simulink model "PeakDetect_500"  (R2018b)
settings: Solver=FixedStepAuto  StartTime=0  StopTime=500*(15e-9)  FixedStep=15e-9  RelTol=1e-3
libraries: simulink x35, hdlsllib x34
(part 1 of 3)
settings Model: FPTRunName=FPA_Reference  Creator=jason  LastModifiedBy=jason
settings OptimizationCC: DefaultParameterBehavior=Inlined

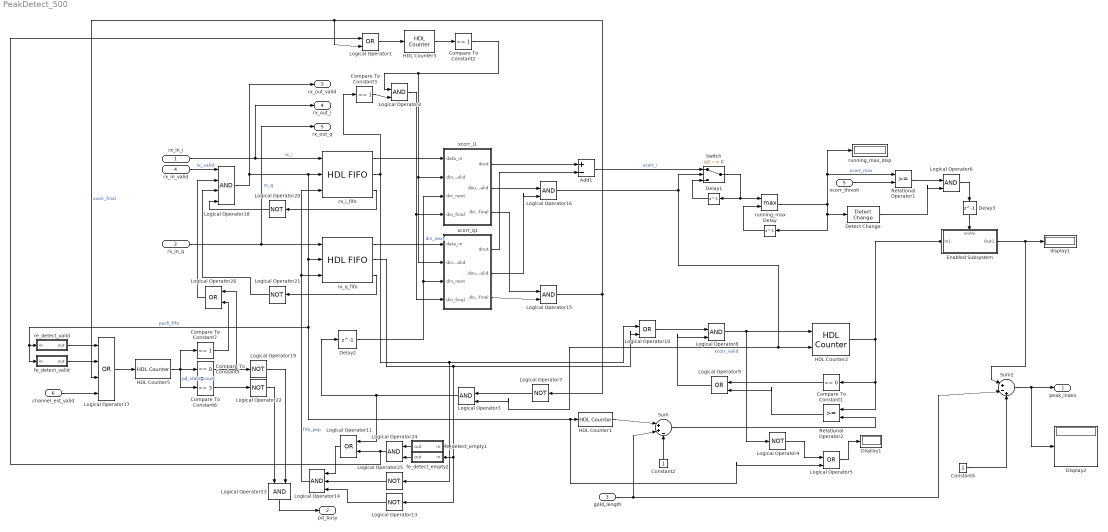
== system PeakDetect_500 ==
  rx_in_i : Inport  OutDataTypeStr=fixdt(1,16,15)  SampleTime=15e-9  Interpolate=off
  rx_in_q : Inport  Port=2  OutDataTypeStr=fixdt(1,16,15)  SampleTime=15e-9  Interpolate=off
  gold_length : Inport  Port=3  OutDataTypeStr=uint16  Interpolate=off
  rx_in_valid : Inport  Port=4  OutDataTypeStr=boolean  SampleTime=15e-9  Interpolate=off
  xcorr_thresh : Inport  Port=5  Interpolate=off
  channel_est_valid : Inport  Port=6  OutDataTypeStr=boolean  Interpolate=off
  Add1 : Sum  Inputs=+-
  Compare To Constant1 : simulink/Logic and Bit Operations/Compare To Constant  relop===  const=0  OutDataTypeStr=boolean
  Compare To Constant2 : simulink/Logic and Bit Operations/Compare To Constant  relop===  const=1  OutDataTypeStr=boolean
  Compare To Constant3 : simulink/Logic and Bit Operations/Compare To Constant  relop===  const=1  OutDataTypeStr=boolean
  Compare To Constant5 : simulink/Logic and Bit Operations/Compare To Constant  relop===  const=0  OutDataTypeStr=boolean
  Compare To Constant6 : simulink/Logic and Bit Operations/Compare To Constant  relop===  const=3  OutDataTypeStr=boolean
  Compare To Constant7 : simulink/Logic and Bit Operations/Compare To Constant  relop===  const=1  OutDataTypeStr=boolean
  Constant2 : Constant  OutDataTypeStr=uint8  SampleTime=-1
  Constant4 : Constant  OutDataTypeStr=uint16  SampleTime=-1
  Delay{,1..3} (4 alike) : Delay  DelayLength=1
  Detect Change : simulink/Logic and Bit Operations/Detect Change  vinit=0  OutDataTypeStr=boolean
  Display1 : Display
  Display2 : Display
  Enabled Subsystem : Subsystem  TreatAsAtomicUnit=on
  HDL Counter1 : hdlsllib/Sources/HDL Counter  CountType=Free running  CountInit=0  CountStep=1  CountMax=25  CountFromType=Initial value  CountFrom=0  CountResetPort=off  CountLoadPort=off  CountEnbPort=on  CountDirPort=off  CountDataType=Unsigned  CountWordLen=16  CountFracLen=0  CountSampTime=1
      settings: SourceProductBaseCode=HD
  HDL Counter2 : hdlsllib/Sources/HDL Counter  CountType=Free running  CountInit=0  CountStep=1  CountMax=25  CountFromType=Initial value  CountFrom=0  CountResetPort=on  CountLoadPort=off  CountEnbPort=on  CountDirPort=off  CountDataType=Unsigned  CountWordLen=16  CountFracLen=0  CountSampTime=1
      settings: SourceProductBaseCode=HD
  HDL Counter3 : hdlsllib/Sources/HDL Counter  CountType=Count limited  CountInit=0  CountStep=1  CountMax=1  CountFromType=Initial value  CountFrom=0  CountResetPort=off  CountLoadPort=off  CountEnbPort=on  CountDirPort=off  CountDataType=Unsigned  CountWordLen=4  CountFracLen=0  CountSampTime=1
      settings: SourceProductBaseCode=HD
  HDL Counter5 : hdlsllib/Sources/HDL Counter  CountType=Count limited  CountInit=0  CountStep=1  CountMax=3  CountFromType=Initial value  CountFrom=0  CountResetPort=off  CountLoadPort=off  CountEnbPort=on  CountDirPort=off  CountDataType=Unsigned  CountWordLen=4  CountFracLen=0  CountSampTime=1
      settings: SourceProductBaseCode=HD
  Logical Operator{1,5,9..11,26} (6 alike) : Logic  Operator=OR  IconShape=distinctive  AllPortsSameDT=off  OutDataTypeStr=boolean
  Logical Operator{4,7,13,19..22,25} (8 alike) : Logic  Operator=NOT  IconShape=distinctive  AllPortsSameDT=off  OutDataTypeStr=boolean
  Logical Operator14 : Logic  Inputs=3  IconShape=distinctive  AllPortsSameDT=off  OutDataTypeStr=boolean
  Logical Operator{2..3,6,8,15..16,23..24} (8 alike) : Logic  IconShape=distinctive  AllPortsSameDT=off  OutDataTypeStr=boolean
  Logical Operator17 : Logic  Operator=OR  Inputs=4  IconShape=distinctive  AllPortsSameDT=off  OutDataTypeStr=boolean
  Logical Operator18 : Logic  Inputs=4  IconShape=distinctive  AllPortsSameDT=off  OutDataTypeStr=boolean
  Relational Operator1 : RelationalOperator  OutDataTypeStr=boolean  RndMeth=Nearest
  Relational Operator2 : RelationalOperator  OutDataTypeStr=boolean  RndMeth=Nearest
  Sum : Sum  Inputs=|++-  AccumDataTypeStr=uint16
  Sum2 : Sum  Inputs=|+-+  AccumDataTypeStr=uint16
  Switch : Switch  Criteria=u2 ~= 0
  display1 : Display
  fe_detect_empty1 : Subsystem
  fe_detect_empty2 : Subsystem
  fe_detect_valid : Subsystem
  re_detect_valid : Subsystem
  running_max : MinMax  Function=max  Inputs=2
  running_max_disp : Display
  rx_i_fifo : hdlsllib/HDL RAMs/HDL FIFO  fifo_size=1024  ratio=1  push_msg=Warning  pop_msg=Warning  show_empty=on  show_full=on  show_num=off
      settings: SourceProductName=HDL Coder  SourceProductBaseCode=HD
  rx_q_fifo : hdlsllib/HDL RAMs/HDL FIFO  fifo_size=1024  ratio=1  push_msg=Warning  pop_msg=Warning  show_empty=on  show_full=on  show_num=off
      settings: SourceProductName=HDL Coder  SourceProductBaseCode=HD
  xcorr_i1 : Subsystem
  xcorr_q1 : Subsystem
  peak_index : Outport  OutDataTypeStr=uint16
  pd_busy : Outport  Port=2
  rx_out_valid : Outport  Port=3  SampleTime=15e-9
  rx_out_i : Outport  Port=4  SampleTime=15e-9
  rx_out_q : Outport  Port=5  SampleTime=15e-9
  wires:
  rx_in_i/1 -> rx_i_fifo/1, rx_out_i/1  "rx_i"
  Add1/1 -> Switch/1  "xcorr_i"
  Enabled Subsystem/1(Out1) -> display1/1, Sum2/1
  gold_length/1 -> Sum2/2, Sum/2
  Sum2/1 -> Display2/1, peak_index/1
  running_max/1 -> Relational Operator1/1, running_max_disp/1, Detect Change/1, Delay/1  "xcorr_max"
  Delay/1 -> running_max/2
  rx_in_q/1 -> rx_q_fifo/1, rx_out_q/1  "rx_q"
  rx_q_fifo/1 -> xcorr_q1/1(data_in)
  rx_i_fifo/2 -> Compare To Constant3/1, Logical Operator25/1, fe_detect_empty1/1(in), Logical Operator10/1
  rx_q_fifo/2 -> fe_detect_empty2/1(in), Logical Operator13/1, Logical Operator10/2
  Sum/1 -> Relational Operator2/2
  HDL Counter1/1 -> Sum/1
  Constant2/1 -> Sum/3
  Constant4/1 -> Sum2/3
  Logical Operator4/1 -> Logical Operator5/1
  Logical Operator5/1 -> Display1/1
  xcorr_thresh/1 -> Relational Operator1/2
  Relational Operator1/1 -> Logical Operator6/1
  Detect Change/1 -> Logical Operator6/2
  xcorr_i1/1(dout) -> Add1/1
  xcorr_q1/1(dout) -> Add1/2
  Logical Operator16/1 -> HDL Counter2/2, Logical Operator3/2, Switch/2  "xcorr_valid"
  HDL Counter2/1 -> Relational Operator2/1, Compare To Constant1/1, Enabled Subsystem/1(In1)
  Compare To Constant1/1 -> Logical Operator9/1
  Relational Operator2/1 -> Logical Operator9/2
  Logical Operator9/1 -> Logical Operator8/2
  Logical Operator8/1 -> Logical Operator4/1, HDL Counter2/1
  Logical Operator10/1 -> Logical Operator8/1
  Logical Operator3/1 -> Delay2/1, Logical Operator11/1
  Delay2/1 -> xcorr_i1/3(din_next), xcorr_q1/3(din_next)  "din_next"
  rx_i_fifo/1 -> xcorr_i1/1(data_in)
  Logical Operator6/1 -> Delay3/1
  Delay3/1 -> Enabled Subsystem/Enable
  HDL Counter3/1 -> Compare To Constant2/1
  Compare To Constant2/1 -> xcorr_i1/2(din_valid), xcorr_q1/2(din_valid), Logical Operator2/1
  Logical Operator24/1 -> Logical Operator1/1, Logical Operator11/2
  Logical Operator1/1 -> HDL Counter3/1
  Logical Operator15/1 -> Logical Operator7/1, Logical Operator17/3, Logical Operator1/2  "xcorr_final"
  Compare To Constant3/1 -> Logical Operator2/2
  Logical Operator2/1 -> xcorr_q1/4(din_final), xcorr_i1/4(din_final)
  Logical Operator7/1 -> Logical Operator3/1
  Logical Operator13/1 -> Logical Operator14/3
  Logical Operator11/1 -> Logical Operator14/1
  Logical Operator14/1 -> rx_i_fifo/3, rx_q_fifo/3  "fifo_pop"
  xcorr_i1/3(dout_final) -> Logical Operator15/1
  xcorr_q1/3(dout_final) -> Logical Operator15/2
  xcorr_q1/2(dout_valid) -> Logical Operator16/2
  xcorr_i1/2(dout_valid) -> Logical Operator16/1
  Logical Operator18/1 -> rx_out_valid/1, rx_q_fifo/2, Logical Operator5/2, HDL Counter1/1, fe_detect_valid/1(in), re_detect_valid/1(in), rx_i_fifo/2  "push_fifo"
  re_detect_valid/1(out) -> Logical Operator17/1
  fe_detect_valid/1(out) -> Logical Operator17/2
  Logical Operator17/1 -> HDL Counter5/1
  channel_est_valid/1 -> Logical Operator17/4
  HDL Counter5/1 -> Compare To Constant7/1, Compare To Constant6/1, Compare To Constant5/1  "pd_state_count"
  rx_in_valid/1 -> Logical Operator18/1  "rx_valid"
  rx_i_fifo/3 -> Logical Operator20/1
  rx_q_fifo/3 -> Logical Operator21/1
  Logical Operator21/1 -> Logical Operator18/3
  Logical Operator20/1 -> Logical Operator18/4
  Compare To Constant5/1 -> Logical Operator26/1, Logical Operator19/1
  Compare To Constant6/1 -> Logical Operator22/1
  Logical Operator22/1 -> Logical Operator23/1
  Logical Operator19/1 -> Logical Operator23/2
  Logical Operator23/1 -> pd_busy/1
  fe_detect_empty1/1(out) -> Logical Operator24/1
  fe_detect_empty2/1(out) -> Logical Operator24/2
  Logical Operator25/1 -> Logical Operator14/2
  Logical Operator26/1 -> Logical Operator18/2
  Compare To Constant7/1 -> Logical Operator26/2
  Switch/1 -> Delay1/1, running_max/1
  Delay1/1 -> Switch/3

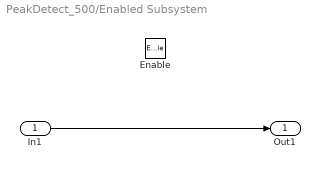
== system PeakDetect_500/Enabled Subsystem ==
  In1 : Inport
  Enable : EnablePort
  Out1 : Outport  InitialOutput=0
  wires:
  In1/1 -> Out1/1

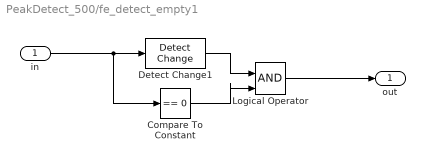
== system PeakDetect_500/fe_detect_empty1 ==
  in : Inport  OutDataTypeStr=boolean
  Compare To Constant : simulink/Logic and Bit Operations/Compare To Constant  relop===  const=0  OutDataTypeStr=boolean
  Detect Change1 : simulink/Logic and Bit Operations/Detect Change  vinit=0  OutDataTypeStr=boolean
  Logical Operator : Logic  IconShape=distinctive  AllPortsSameDT=off  OutDataTypeStr=boolean
  out : Outport  OutDataTypeStr=boolean
  wires:
  Logical Operator/1 -> out/1
  Detect Change1/1 -> Logical Operator/1
  Compare To Constant/1 -> Logical Operator/2
  in/1 -> Compare To Constant/1, Detect Change1/1

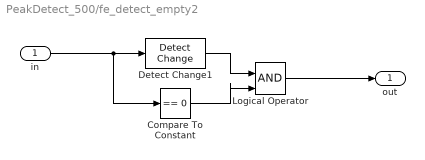
== system PeakDetect_500/fe_detect_empty2 ==
  in : Inport  OutDataTypeStr=boolean
  Compare To Constant : simulink/Logic and Bit Operations/Compare To Constant  relop===  const=0  OutDataTypeStr=boolean
  Detect Change1 : simulink/Logic and Bit Operations/Detect Change  vinit=0  OutDataTypeStr=boolean
  Logical Operator : Logic  IconShape=distinctive  AllPortsSameDT=off  OutDataTypeStr=boolean
  out : Outport  OutDataTypeStr=boolean
  wires:
  Logical Operator/1 -> out/1
  Detect Change1/1 -> Logical Operator/1
  Compare To Constant/1 -> Logical Operator/2
  in/1 -> Compare To Constant/1, Detect Change1/1

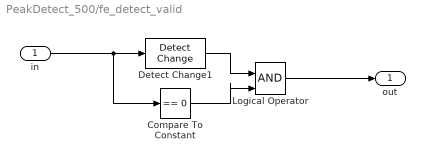
== system PeakDetect_500/fe_detect_valid ==
  in : Inport  OutDataTypeStr=boolean
  Compare To Constant : simulink/Logic and Bit Operations/Compare To Constant  relop===  const=0  OutDataTypeStr=boolean
  Detect Change1 : simulink/Logic and Bit Operations/Detect Change  vinit=0  OutDataTypeStr=boolean
  Logical Operator : Logic  IconShape=distinctive  AllPortsSameDT=off  OutDataTypeStr=boolean
  out : Outport  OutDataTypeStr=boolean
  wires:
  Logical Operator/1 -> out/1
  Detect Change1/1 -> Logical Operator/1
  Compare To Constant/1 -> Logical Operator/2
  in/1 -> Compare To Constant/1, Detect Change1/1

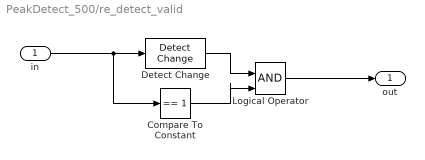
== system PeakDetect_500/re_detect_valid ==
  in : Inport  OutDataTypeStr=boolean
  Compare To Constant : simulink/Logic and Bit Operations/Compare To Constant  relop===  const=1  OutDataTypeStr=boolean
  Detect Change : simulink/Logic and Bit Operations/Detect Change  vinit=0  OutDataTypeStr=boolean
  Logical Operator : Logic  IconShape=distinctive  AllPortsSameDT=off  OutDataTypeStr=boolean
  out : Outport  OutDataTypeStr=boolean
  wires:
  Logical Operator/1 -> out/1
  Compare To Constant/1 -> Logical Operator/2
  Detect Change/1 -> Logical Operator/1
  in/1 -> Compare To Constant/1, Detect Change/1

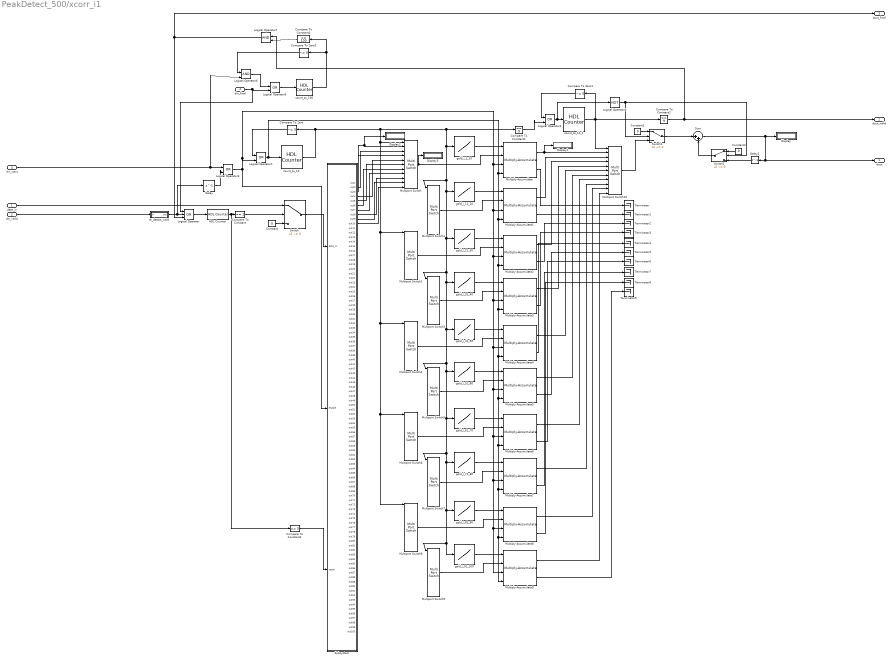
== system PeakDetect_500/xcorr_i1 ==
  data_in : Inport  OutDataTypeStr=fixdt(1,16,15)
  din_valid : Inport  Port=2
  din_next : Inport  Port=3
  din_final : Inport  Port=4
  Compare To Constant : simulink/Logic and Bit Operations/Compare To Constant  relop===  const=1  OutDataTypeStr=boolean
  Compare To Constant1 : simulink/Logic and Bit Operations/Compare To Constant  relop===  const=9  OutDataTypeStr=boolean
  Compare To Constant2 : simulink/Logic and Bit Operations/Compare To Constant  relop===  const=9  OutDataTypeStr=boolean
  Compare To Constant3 : simulink/Logic and Bit Operations/Compare To Constant  relop===  const=100  OutDataTypeStr=boolean
  Compare To Constant4 : simulink/Logic and Bit Operations/Compare To Constant  relop===  const=0  OutDataTypeStr=boolean
  Compare To Zero : simulink/Logic and Bit Operations/Compare To Zero  relop=~=  OutDataTypeStr=boolean
  Compare To Zero1 : simulink/Logic and Bit Operations/Compare To Zero  relop=~=  OutDataTypeStr=boolean
  Compare To Zero2 : simulink/Logic and Bit Operations/Compare To Zero  relop=~=  OutDataTypeStr=boolean
  Constant : Constant  Value=0  OutDataTypeStr=fixdt(1,16,15)  SampleTime=-1
  Constant1 : Constant  Value=0  OutDataTypeStr=Inherit: Inherit via back propagation  SampleTime=-1
  Constant2 : Constant  Value=0  OutDataTypeStr=Inherit: Inherit via back propagation  SampleTime=-1
  Delay : Delay  DelayLength=1
  Delay2 : Delay  DelayLength=1
  Display{,1..3} (4 alike) : Display
  HDL Counter : hdlsllib/Sources/HDL Counter  CountType=Count limited  CountInit=0  CountStep=1  CountMax=2  CountFromType=Initial value  CountFrom=0  CountResetPort=off  CountLoadPort=off  CountEnbPort=on  CountDirPort=off  CountDataType=Unsigned  CountWordLen=8  CountFracLen=0  CountSampTime=1
      settings: SourceProductBaseCode=HD
  Logical Operator : Logic  Operator=OR  Inputs=3  IconShape=distinctive  AllPortsSameDT=off  OutDataTypeStr=boolean
  Logical Operator{1..3,5} (4 alike) : Logic  Operator=OR  IconShape=distinctive  AllPortsSameDT=off  OutDataTypeStr=boolean
  Logical Operator4 : Logic  Operator=NOT  IconShape=distinctive  AllPortsSameDT=off  OutDataTypeStr=boolean
  Logical Operator6 : Logic  IconShape=distinctive  AllPortsSameDT=off  OutDataTypeStr=boolean
  Logical Operator7 : Logic  IconShape=distinctive  AllPortsSameDT=off  OutDataTypeStr=boolean
  Multiply-Accumulate{,1..9} (10 alike) : hdlsllib/HDL Operations/Multiply-Accumulate  opMode=Streaming - using Start and End ports  initValueSetting=Dialog  initValue=0  initValueSetting2=Dialog  initValue2=0  initValueSetting3=Dialog  initValue3=0  num_samples=2  RndMeth2=Floor  RndMeth3=Floor  datatype2=fixdt(1,32,16)  datatype3=Inherit: Inherit via back propagation  validOut=on  endInandOut=off  startOut=off  countOut=on  dim=-1  DoSatur=off  parallel=off
      settings: SourceProductName=HDL Coder  SourceProductBaseCode=HD
  Multiport Switch{,1..9} (10 alike) : MultiPortSwitch  DataPortOrder=Zero-based contiguous  Inputs=10  zeroidx=on  OutDataTypeStr=fixdt(1,16,15)
  Multiport Switch10 : MultiPortSwitch  DataPortOrder=Zero-based contiguous  Inputs=10  zeroidx=on  OutDataTypeStr=fixdt(1,32,16)
  Subsystem : Subsystem
  Sum : Sum  Inputs=|++  OutDataTypeStr=Inherit: Inherit via back propagation
  Switch : Switch  Criteria=u2 ~= 0  OutDataTypeStr=Inherit: Inherit via back propagation
  Switch1 : Switch  Criteria=u2 ~= 0  OutDataTypeStr=Inherit: Inherit via back propagation
  Switch2 : Switch  Criteria=u2 ~= 0  OutDataTypeStr=Inherit: Inherit via back propagation
  Terminator{,1..9} (10 alike) : Terminator
  count_to_10 : hdlsllib/Sources/HDL Counter  CountType=Count limited  CountInit=0  CountStep=1  CountMax=9  CountFromType=Initial value  CountFrom=0  CountResetPort=off  CountLoadPort=off  CountEnbPort=on  CountDirPort=off  CountDataType=Unsigned  CountWordLen=4  CountFracLen=0  CountSampTime=1
      settings: SourceProductBaseCode=HD
  count_to_100 : hdlsllib/Sources/HDL Counter  CountType=Count limited  CountInit=0  CountStep=1  CountMax=100  CountFromType=Initial value  CountFrom=0  CountResetPort=off  CountLoadPort=off  CountEnbPort=on  CountDirPort=off  CountDataType=Unsigned  CountWordLen=8  CountFracLen=0  CountSampTime=1
      settings: SourceProductBaseCode=HD
  count_to_10_2 : hdlsllib/Sources/HDL Counter  CountType=Count limited  CountInit=0  CountStep=1  CountMax=9  CountFromType=Initial value  CountFrom=0  CountResetPort=off  CountLoadPort=off  CountEnbPort=on  CountDirPort=off  CountDataType=Unsigned  CountWordLen=4  CountFracLen=0  CountSampTime=1
      settings: SourceProductBaseCode=HD
  gold_i_11_20 : Lookup_n-D  NumberOfTableDimensions=1  LookupTableObject=''  BreakpointsForDimension1=uint8([0,1,2,3,4,5,6,7,8,9])  BreakpointsForDimension1FirstPoint=10  BreakpointsForDimension2FirstPoint=10  BreakpointsForDimension1Spacing=12  BreakpointsForDimension2Spacing=12  IndexSearchMethod=Evenly spaced points  Table=|  TableDataTypeStr=fixdt(1,16,15)  InterpMethod=Flat  DiagnosticForOutOfRangeInput=Error  InternalRulePriority=Speed  OutDataTypeStr=fixdt(1,16,15)  RndMeth=Simplest  InputSameDT=on
      | [0.236906374990369
      | 0.265062589296935
      | 0.290853922757752
      | 0.306866645010829
      | 0.306877356493505
      | 0.282583044796408
      | 0.237895318583737
      | 0.179451570247324
      | 0.106711739895776
      | 0.0250742736874029]
  gold_i_1_10 : Lookup_n-D  NumberOfTableDimensions=1  LookupTableObject=''  BreakpointsForDimension1=uint8([0,1,2,3,4,5,6,7,8,9])  BreakpointsForDimension1FirstPoint=10  BreakpointsForDimension2FirstPoint=10  BreakpointsForDimension1Spacing=12  BreakpointsForDimension2Spacing=12  IndexSearchMethod=Evenly spaced points  Table=|  TableDataTypeStr=fixdt(1,16,15)  InterpMethod=Flat  DiagnosticForOutOfRangeInput=Error  InternalRulePriority=Speed  OutDataTypeStr=fixdt(1,16,15)  RndMeth=Simplest  InputSameDT=on
      | [0.357169275362262
      | 0.373691122276015
      | 0.363136475782144
      | 0.332586509539436
      | 0.291374087870011
      | 0.249422279627694
      | 0.215579045674242
      | 0.200455944131648
      | 0.201796906991478
      | 0.213779029408702]
  gold_i_21_30 : Lookup_n-D  NumberOfTableDimensions=1  LookupTableObject=''  BreakpointsForDimension1=uint8([0,1,2,3,4,5,6,7,8,9])  BreakpointsForDimension1FirstPoint=10  BreakpointsForDimension2FirstPoint=10  BreakpointsForDimension1Spacing=12  BreakpointsForDimension2Spacing=12  IndexSearchMethod=Evenly spaced points  Table=|  TableDataTypeStr=fixdt(1,16,15)  InterpMethod=Flat  DiagnosticForOutOfRangeInput=Error  InternalRulePriority=Speed  OutDataTypeStr=fixdt(1,16,15)  RndMeth=Simplest  InputSameDT=on
      | [-0.0591515848508664
      | -0.139598314313151
      | -0.210629837752387
      | -0.263713716480122
      | -0.301489962058033
      | -0.328238114626508
      | -0.340130412877520
      | -0.338689881672749
      | -0.326243180584237
      | -0.305614110780615]
  gold_i_31_40 : Lookup_n-D  NumberOfTableDimensions=1  LookupTableObject=''  BreakpointsForDimension1=uint8([0,1,2,3,4,5,6,7,8,9])  BreakpointsForDimension1FirstPoint=10  BreakpointsForDimension2FirstPoint=10  BreakpointsForDimension1Spacing=12  BreakpointsForDimension2Spacing=12  IndexSearchMethod=Evenly spaced points  Table=|  TableDataTypeStr=fixdt(1,16,15)  InterpMethod=Flat  DiagnosticForOutOfRangeInput=Error  InternalRulePriority=Speed  OutDataTypeStr=fixdt(1,16,15)  RndMeth=Simplest  InputSameDT=on
      | [-0.279858098355888
      | -0.247814863771713
      | -0.225446174923891
      | -0.202743193363060
      | -0.186527042991191
      | -0.178781266249413
      | -0.180711431323688
      | -0.192575241083779
      | -0.213551675353352
      | -0.245925394077466]
  gold_i_41_50 : Lookup_n-D  NumberOfTableDimensions=1  LookupTableObject=''  BreakpointsForDimension1=uint8([0,1,2,3,4,5,6,7,8,9])  BreakpointsForDimension1FirstPoint=10  BreakpointsForDimension2FirstPoint=10  BreakpointsForDimension1Spacing=12  BreakpointsForDimension2Spacing=12  IndexSearchMethod=Evenly spaced points  Table=|  TableDataTypeStr=fixdt(1,16,15)  InterpMethod=Flat  DiagnosticForOutOfRangeInput=Error  InternalRulePriority=Speed  OutDataTypeStr=fixdt(1,16,15)  RndMeth=Simplest  InputSameDT=on
      | [-0.273649789754997
      | -0.305507933389466
      | -0.332526349511340
      | -0.349961882407133
      | -0.353614169955030
      | -0.340366684130075
      | -0.308641627170326
      | -0.254460428744123
      | -0.185247665828561
      | -0.110080691949015]
  gold_i_51_60 : Lookup_n-D  NumberOfTableDimensions=1  LookupTableObject=''  BreakpointsForDimension1=uint8([0,1,2,3,4,5,6,7,8,9])  BreakpointsForDimension1FirstPoint=10  BreakpointsForDimension2FirstPoint=10  BreakpointsForDimension1Spacing=12  BreakpointsForDimension2Spacing=12  IndexSearchMethod=Evenly spaced points  Table=|  TableDataTypeStr=fixdt(1,16,15)  InterpMethod=Flat  DiagnosticForOutOfRangeInput=Error  InternalRulePriority=Speed  OutDataTypeStr=fixdt(1,16,15)  RndMeth=Simplest  InputSameDT=on
      | [-0.0297558495000080
      | 0.0499350486257353
      | 0.122950591883728
      | 0.183532283875116
      | 0.226715241693549
      | 0.244522518247979
      | 0.247772413924009
      | 0.223279362418140
      | 0.176793915855740
      | 0.111355596734925]
  gold_i_61_70 : Lookup_n-D  NumberOfTableDimensions=1  LookupTableObject=''  BreakpointsForDimension1=uint8([0,1,2,3,4,5,6,7,8,9])  BreakpointsForDimension1FirstPoint=10  BreakpointsForDimension2FirstPoint=10  BreakpointsForDimension1Spacing=12  BreakpointsForDimension2Spacing=12  IndexSearchMethod=Evenly spaced points  Table=|  TableDataTypeStr=fixdt(1,16,15)  InterpMethod=Flat  DiagnosticForOutOfRangeInput=Error  InternalRulePriority=Speed  OutDataTypeStr=fixdt(1,16,15)  RndMeth=Simplest  InputSameDT=on
      | [0.0312880626224120
      | -0.0580988665112754
      | -0.150830519884918
      | -0.236354458852815
      | -0.321361371110983
      | -0.387151947785857
      | -0.432910784333285
      | -0.454553321854592
      | -0.449340647995132
      | -0.416266380216616]
  gold_i_71_80 : Lookup_n-D  NumberOfTableDimensions=1  LookupTableObject=''  BreakpointsForDimension1=uint8([0,1,2,3,4,5,6,7,8,9])  BreakpointsForDimension1FirstPoint=10  BreakpointsForDimension2FirstPoint=10  BreakpointsForDimension1Spacing=12  BreakpointsForDimension2Spacing=12  IndexSearchMethod=Evenly spaced points  Table=|  TableDataTypeStr=fixdt(1,16,15)  InterpMethod=Flat  DiagnosticForOutOfRangeInput=Error  InternalRulePriority=Speed  OutDataTypeStr=fixdt(1,16,15)  RndMeth=Simplest  InputSameDT=on
      | [-0.356405677154333
      | -0.268905527196357
      | -0.172503144328213
      | -0.0623088722264564
      | 0.0478292512438747
      | 0.147701871156711
      | 0.227579808283800
      | 0.279365016179912
      | 0.297653875710057
      | 0.276310228166542]
  gold_i_81_90 : Lookup_n-D  NumberOfTableDimensions=1  LookupTableObject=''  BreakpointsForDimension1=uint8([0,1,2,3,4,5,6,7,8,9])  BreakpointsForDimension1FirstPoint=10  BreakpointsForDimension2FirstPoint=10  BreakpointsForDimension1Spacing=12  BreakpointsForDimension2Spacing=12  IndexSearchMethod=Evenly spaced points  Table=|  TableDataTypeStr=fixdt(1,16,15)  InterpMethod=Flat  DiagnosticForOutOfRangeInput=Error  InternalRulePriority=Speed  OutDataTypeStr=fixdt(1,16,15)  RndMeth=Simplest  InputSameDT=on
      | [0.222595237130309
      | 0.147485843722747
      | 0.0555170073150737
      | -0.0424496465550990
      | -0.134707118174198
      | -0.210100315272752
      | -0.259403813850479
      | -0.272248751146779
      | -0.259403813850479
      | -0.210100315272752]
  gold_i_91_100 : Lookup_n-D  NumberOfTableDimensions=1  LookupTableObject=''  BreakpointsForDimension1=uint8([0,1,2,3,4,5,6,7,8,9])  BreakpointsForDimension1FirstPoint=10  BreakpointsForDimension2FirstPoint=10  BreakpointsForDimension1Spacing=12  BreakpointsForDimension2Spacing=12  IndexSearchMethod=Evenly spaced points  Table=|  TableDataTypeStr=fixdt(1,16,15)  InterpMethod=Flat  DiagnosticForOutOfRangeInput=Error  InternalRulePriority=Speed  OutDataTypeStr=fixdt(1,16,15)  RndMeth=Simplest  InputSameDT=on
      | [-0.134707118174198
      | -0.0424496465550990
      | 0.0555170073150737
      | 0.147485843722747
      | 0.222595237130309
      | 0.267820298855522
      | 0.290378842162360
      | 0.275261187855880
      | 0.228204197191429
      | 0.153805243290024]
  re_detect_valid : Subsystem
  dout : Outport  OutDataTypeStr=fixdt(1,32,16)
  dout_valid : Outport  Port=2
  dout_final : Outport  Port=3
  wires:
  ? -> Multiport Switch3/4
  Compare To Constant2/1 -> dout_valid/1, Logical Operator7/1
  ? -> Multiport Switch4/6
  ? -> Multiport Switch1/8
  Logical Operator1/1 -> count_to_10/1, Multiply-Accumulate2/4, Multiply-Accumulate9/4, Multiply-Accumulate8/4, Multiply-Accumulate7/4, Multiply-Accumulate6/4, Multiply-Accumulate5/4, Multiply-Accumulate4/4, Multiply-Accumulate3/4, Multiply-Accumulate1/4, Multiply-Accumulate/4
  gold_i_21_30/1 -> Multiply-Accumulate2/1
  HDL Counter/1 -> Compare To Constant4/1, Compare To Constant/1
  count_to_100/1 -> Compare To Constant3/1, Compare To Zero2/1
  Subsystem/5(out5) -> Multiport Switch/6
  Logical Operator3/1 -> Subsystem/2(enable), Multiply-Accumulate9/3, Multiply-Accumulate8/3, Multiply-Accumulate7/3, Multiply-Accumulate6/3, Multiply-Accumulate5/3, Multiply-Accumulate4/3, Multiply-Accumulate3/3, Multiply-Accumulate2/3, Multiply-Accumulate1/3, Multiply-Accumulate/3, Logical Operator1/2
  Constant2/1 -> Switch2/1
  ? -> Multiport Switch7/10
  din_next/1 -> Logical Operator6/2, Logical Operator3/1
  Subsystem/6(out6) -> Multiport Switch/7
  ? -> Multiport Switch2/9
  count_to_10/1 -> Compare To Zero/1, Multiport Switch8/1, Multiport Switch6/1, Multiport Switch4/1, Multiport Switch2/1, Multiport Switch/1, gold_i_11_20/1, gold_i_21_30/1, gold_i_31_40/1, gold_i_41_50/1, gold_i_51_60/1, gold_i_61_70/1, gold_i_71_80/1, gold_i_81_90/1, gold_i_91_100/1, Multiport Switch9/1, Multiport Switch7/1, Multiport Switch5/1, Multiport Switch3/1, Multiport Switch1/1, gold_i_1_10/1, Compare To Constant1/1
  Multiport Switch10/1 -> Switch1/3
  Logical Operator4/1 -> Switch2/2, Switch1/2
  Constant/1 -> Switch/3
  ? -> Multiport Switch4/7
  ? -> Multiport Switch9/2
  ? -> Multiport Switch5/5
  Compare To Constant4/1 -> Subsystem/3(reset)
  ? -> Multiport Switch5/4
  Logical Operator6/1 -> Logical Operator5/1
  Sum/1 -> dout/1, Delay2/1, Display/1
  ? -> Multiport Switch3/5
  ? -> Multiport Switch3/9
  Multiport Switch2/1 -> Multiply-Accumulate2/2
  Multiply-Accumulate6/2 -> Terminator6/1
  data_in/1 -> Switch/1
  Logical Operator2/1 -> Logical Operator4/1, count_to_10_2/1
  Subsystem/8(out8) -> Multiport Switch/9
  Delay2/1 -> Switch2/3
  ? -> Multiport Switch4/5
  Logical Operator7/1 -> dout_final/1, Logical Operator/3
  ? -> Multiport Switch2/5
  Multiply-Accumulate9/2 -> Terminator9/1
  ? -> Multiport Switch3/7
  ? -> Multiport Switch8/2
  ? -> Multiport Switch1/3
  Switch2/1 -> Sum/2
  re_detect_valid/1(out) -> Logical Operator/2, Delay/1
  Multiport Switch5/1 -> Multiply-Accumulate5/2
  ? -> Multiport Switch4/3
  ? -> Multiport Switch2/7
  count_to_10_2/1 -> Compare To Constant2/1, Multiport Switch10/1, Compare To Zero1/1
  ? -> Multiport Switch9/5
  ? -> Multiport Switch3/11
  ? -> Multiport Switch4/8
  ? -> Multiport Switch4/4
  Logical Operator5/1 -> count_to_100/1
  ? -> Multiport Switch5/7
  ? -> Multiport Switch6/6
  Switch1/1 -> Sum/1
  ? -> Multiport Switch3/6
  ? -> Multiport Switch9/11
  Compare To Constant/1 -> Switch/2
  ? -> Multiport Switch9/7
  ? -> Multiport Switch4/9
  ? -> Multiport Switch2/4
  Multiply-Accumulate4/2 -> Terminator4/1
  ? -> Multiport Switch7/4
  ? -> Multiport Switch5/10
  Multiply-Accumulate7/2 -> Terminator7/1
  Multiport Switch3/1 -> Multiply-Accumulate3/2
  ? -> Multiport Switch2/10
  ? -> Multiport Switch1/7
  Compare To Zero2/1 -> Logical Operator6/1
  ? -> Multiport Switch9/3
  ? -> Multiport Switch3/8
  ? -> Multiport Switch6/7
  gold_i_61_70/1 -> Multiply-Accumulate6/1
  ? -> Multiport Switch5/11
  Multiply-Accumulate3/2 -> Terminator3/1
  Switch/1 -> Subsystem/1(data_in)
  ? -> Multiport Switch9/10
  Delay/1 -> Logical Operator3/2
  Multiply-Accumulate5/2 -> Terminator5/1
  Subsystem/7(out7) -> Multiport Switch/8
  ? -> Multiport Switch4/10
  ? -> Multiport Switch3/3
  Compare To Zero/1 -> Logical Operator1/1
  gold_i_81_90/1 -> Multiply-Accumulate8/1
  ? -> Multiport Switch8/5
  ? -> Multiport Switch9/9
  gold_i_1_10/1 -> Multiply-Accumulate/1
  Multiport Switch1/1 -> Multiply-Accumulate1/2
  Multiport Switch4/1 -> Multiply-Accumulate4/2
  ? -> Multiport Switch8/11
  ? -> Multiport Switch2/2
  gold_i_41_50/1 -> Multiply-Accumulate4/1
  gold_i_51_60/1 -> Multiply-Accumulate5/1
  Multiport Switch7/1 -> Multiply-Accumulate7/2
  ? -> Multiport Switch2/8
  ? -> Multiport Switch5/2
  ? -> Multiport Switch7/11
  ? -> Multiport Switch5/8
  ? -> Multiport Switch3/2
  ? -> Multiport Switch6/2
  ? -> Multiport Switch6/9
  ? -> Multiport Switch6/3
  ? -> Multiport Switch6/4
  ? -> Multiport Switch6/10
  Compare To Constant1/1 -> Logical Operator2/2
  Subsystem/9(out9) -> Multiport Switch/10
  ? -> Multiport Switch4/11
  ? -> Multiport Switch5/6
  ? -> Multiport Switch7/3
  ? -> Multiport Switch7/8
  ? -> Multiport Switch7/5
  Multiport Switch/1 -> Multiply-Accumulate/2, Display3/1
  ? -> Multiport Switch2/6
  ? -> Multiport Switch7/6
  ? -> Multiport Switch7/9
  ? -> Multiport Switch2/11
  ? -> Multiport Switch4/2
  ? -> Multiport Switch8/3
  ? -> Multiport Switch8/6
  Subsystem/2(out2) -> Multiport Switch/3
  ? -> Multiport Switch8/8
  ? -> Multiport Switch8/4
  ? -> Multiport Switch8/7
  ? -> Multiport Switch9/6
  ? -> Multiport Switch8/9
  ? -> Multiport Switch1/11
  ? -> Multiport Switch8/10
  ? -> Multiport Switch1/10
  Compare To Constant3/1 -> Logical Operator7/2
  ? -> Multiport Switch3/10
  Multiply-Accumulate8/1 -> Multiport Switch10/10
  Multiply-Accumulate7/1 -> Multiport Switch10/9
  ? -> Multiport Switch9/8
  Multiply-Accumulate6/1 -> Multiport Switch10/8
  gold_i_31_40/1 -> Multiply-Accumulate3/1
  Multiport Switch8/1 -> Multiply-Accumulate8/2
  Multiply-Accumulate5/1 -> Multiport Switch10/7
  gold_i_11_20/1 -> Multiply-Accumulate1/1
  din_final/1 -> Logical Operator/1, Logical Operator5/2
  gold_i_71_80/1 -> Multiply-Accumulate7/1
  ? -> Multiport Switch5/3
  ? -> Multiport Switch1/9
  Multiport Switch6/1 -> Multiply-Accumulate6/2
  Subsystem/10(out10) -> Multiport Switch/11
  Multiply-Accumulate9/1 -> Multiport Switch10/11
  ? -> Multiport Switch6/8
  ? -> Multiport Switch7/7
  Multiply-Accumulate3/1 -> Multiport Switch10/5
  ? -> Multiport Switch5/9
  Constant1/1 -> Switch1/1
  Multiport Switch9/1 -> Multiply-Accumulate9/2
  ? -> Multiport Switch7/2
  ? -> Multiport Switch2/3
  ? -> Multiport Switch1/5
  Multiply-Accumulate/1 -> Display1/1, Multiport Switch10/2
  ? -> Multiport Switch6/5
  ? -> Multiport Switch6/11
  Compare To Zero1/1 -> Logical Operator2/1
  Multiply-Accumulate2/1 -> Multiport Switch10/4
  gold_i_91_100/1 -> Multiply-Accumulate9/1
  Multiply-Accumulate4/1 -> Multiport Switch10/6
  Multiply-Accumulate1/1 -> Multiport Switch10/3
  ? -> Multiport Switch9/4
  Logical Operator/1 -> HDL Counter/1
  ? -> Multiport Switch1/4
  Subsystem/1(out1) -> Multiport Switch/2, Display2/1
  din_valid/1 -> re_detect_valid/1(in)
  ? -> Multiport Switch1/6
  ? -> Multiport Switch1/2
  Subsystem/3(out3) -> Multiport Switch/4
  Subsystem/4(out4) -> Multiport Switch/5
  Multiply-Accumulate/2 -> Terminator/1
  Multiply-Accumulate1/2 -> Terminator1/1
  Multiply-Accumulate2/2 -> Terminator2/1
  Multiply-Accumulate8/2 -> Terminator8/1
